simulink model "animation_wrk"  (R2021b)
settings: Solver=VariableStepAuto  StartTime=0.0  StopTime=t(end)  RelTol=1e-3
libraries: aerolibanim x2, aerolibsim3d x1, sim3dlib x1
settings Model: Creator=schae  LastModifiedBy=schae

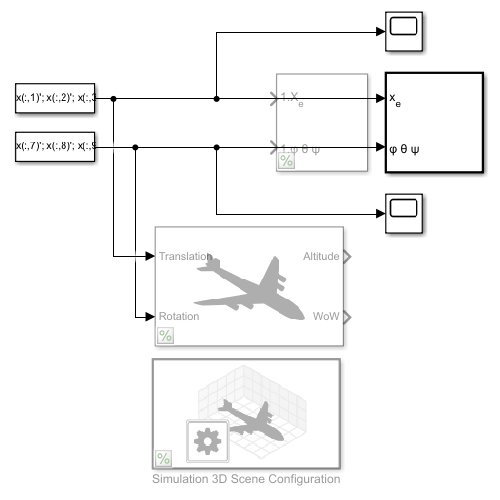
[thumbnail: Simulink's stored preview of the top-level diagram]
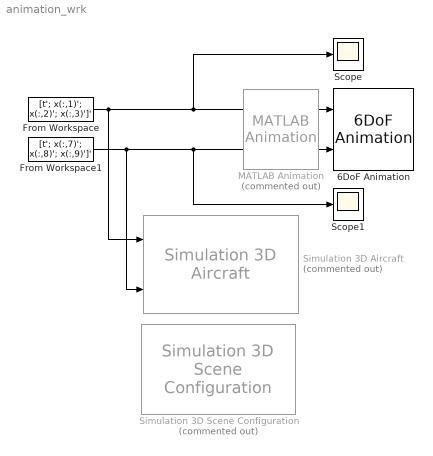
== system animation_wrk ==
  6DoF Animation : aerolibanim/6DoF Animation  u1=[0 15 -5 5 -5 0]  u2=5e-3  u3=0.25  u4=[0 0 -1]  u5=Fixed position  u6=[25 15 -5]  u7=10  u8=on
  From Workspace : FromWorkspace  VariableName=[t'; x(:,1)'; x(:,2)'; x(:,3)']'
  From Workspace1 : FromWorkspace  VariableName=[t'; x(:,7)'; x(:,8)'; x(:,9)']'
  MATLAB Animation : aerolibanim/MATLAB Animation  Tag=Matlab Animation 6 DOF  Commented=on  Vehicles=1  Geometries='astredwedge.mat'  BoundingBoxCoordinates=[-50,50,-50,50,-50,50]  CameraOffset=[-150,-50,0]  CameraViewAngle=3  SampleTime=0.2  FigurePosition=[403,303,275,214]
      settings: SourceProductBaseCode=AE
  Scope : Scope
  Scope1 : Scope
  Simulation 3D Aircraft : aerolibsim3d/Simulation 3D Aircraft  Commented=on  Mesh=SkyHogg  AircraftColor=Red  ActorName=SimulinkVehicle1  Translation=zeros( 11, 3 )  Rotation=zeros( 11, 3 )  IsGHSensorEnabled=on  AreGHRaysVisible=off  GHRayLength=1524  GHBodyOffset=0.90  GHFrontTireRadius=0.21  GHLeftTireRadius=0.21  GHRightTireRadius=0.21  SampleTime=-1  ActorType=SimulinkVehicle  ID=1  aMode=0  ActorTag=SimulinkVehicle1
      settings: SourceProductBaseCode=AE
  Simulation 3D Scene Configuration : sim3dlib/Simulation 3D Scene Configuration  Priority=0  Commented=on  ProjectFormat_internal=Default Scenes  ProjectFormat=Default Scenes  SceneDesc=Airport  ProjectName=C:\Program Files\MATLAB\R2021b\toolbox\shared\sim3d_projects\automotive_project\UE4\WindowsNoEditor\VehicleSimulation.exe  ScenePath=/Game/Maps/HwStrght  vehTagList={'Scene Origin';'SimulinkVehicle1'}  vehTag=SimulinkVehicle1  OpVisEn=off  Ts=.02  EnableWindow=on  EnableWeather=off  SunAltitude=40.0  SunAzimuth=90  clouds=10  wind=1  fog=0  rain=0  sensorTag=MainCamera1  sensorId=1  sensorName=MainCamera1  mountLoc=Origin  offsetFlag=off  tmountOffset=[0, 0, 0]  rmountOffset=[0, 0, 0]  HorizontalResolution=1280  VerticalResolution=720  HorizontalFOV=60  mountPoint=[0 0 0]  mountOrientation=[0 0 0]  aMode=0  ID=1
      settings: SourceProductBaseCode=AE,DR,UV,VE
  wires:
  From Workspace/1 -> Simulation 3D Aircraft/1, 6DoF Animation/1, Scope/1
  From Workspace1/1 -> Simulation 3D Aircraft/2, 6DoF Animation/2, Scope1/1
